simulink model "QPSK_system_v3g"  (R2012b)
settings: Solver=FixedStepDiscrete  SolverMode=SingleTasking  StartTime=0.0  StopTime=6000  FixedStep=1  RelTol=1e-3
libraries: simulink x30, dspsigops x2, dspbuff3 x1, dspsrcs4 x1
(part 4 of 4)

== matlab function QPSK_system_v3g/RX_CORE_TOP/RX/rx_double/qpsk_rx ==
  data: i_in input; byte_out output; q_in input; mu_foc_in input; mu_toc_in input; mcu_rx_ready_in input; en_out output; clear_fifo_out output; num_bytes_ready_out output; r_out output; s_f_out output; s_c_out output; s_t_out output; t_est_out output; s_p_out output; s_o_out output; fe_out output
%%%%%%%%%%%%%%%%%%%%%%%%%%%%%%%%%%%%%%%%%%%%%%%%%%%%%%%%%%%%%%%%%%%%%%%%%%%
% QPSK demonstration packet-based transceiver for Chilipepper
% Toyon Research Corp.
% http://www.toyon.com/chilipepper.php
% Created 10/17/2012
% embedded@toyon.com
%%%%%%%%%%%%%%%%%%%%%%%%%%%%%%%%%%%%%%%%%%%%%%%%%%%%%%%%%%%%%%%%%%%%%%%%%%%
% This file is the top level entry function for the receiver portion of the
% example. The entire receiver is designed to run at Rate=1 (one clock
% cycle per iteration of the core. 
% We follow standard receive practice with frequency offset estimation,
% pulse-shape filtering, time estimateion, and correlation to determine
% tart of packet.
%%%%%%%%%%%%%%%%%%%%%%%%%%%%%%%%%%%%%%%%%%%%%%%%%%%%%%%%%%%%%%%%%%%%%%%%%%%
%#codegen
function [byte_out, en_out, clear_fifo_out, num_bytes_ready_out, ...
        r_out, s_f_out, s_c_out, s_t_out, t_est_out, s_p_out, s_o_out, ...
        fe_out] = ...
    qpsk_rx(i_in, q_in, mu_foc_in, mu_toc_in, mcu_rx_ready_in)

persistent finish_rx_latch

if isempty(finish_rx_latch)
    finish_rx_latch = 0; % feedback once packet is received to rest
end

i_in = round(i_in);
q_in = round(q_in);

% scale input data coming from the Chilipepper ADC to be purely fractional
% to avoid scaling issues
r_in = complex(i_in, q_in);

% frequency offset estimation. Note that time constant is input as integer
[s_f_i, s_f_q, fe] = ...
    qpsk_rx_foc(i_in, q_in, mu_foc_in, finish_rx_latch);

   if finish_rx_latch > 0
    a=0;
   end

% Square-root raised-cosine band-limited filtering
[s_c_i, s_c_q] = qpsk_rx_srrc(s_f_i, s_f_q);

% Time offset estimation. Output data changes at the symbol rate.
[s_t_i, s_t_q, tauh] = ...
    qpsk_rx_toc(s_c_i, s_c_q, mu_toc_in, finish_rx_latch);

% Determine start of packet using front-loaded training sequence
[byte, en, finish_rx, clear_fifo, num_bytes_ready_out, s_p, s_o] = ...
    qpsk_rx_correlator(s_t_i, s_t_q, mcu_rx_ready_in);


% These are debug outputs and can largely be ignored as they are just used
% for testbench simulation
byte_out = byte;
en_out = en;
clear_fifo_out = clear_fifo;

finish_rx_latch = finish_rx;

%r_out = real(r_in);
r_out = r_in;
s_f_out = complex(s_f_i,s_f_q);
s_c_out = complex(s_c_i,s_c_q);
s_t_out = complex(s_t_i,s_t_q);

t_est_out = tauh;
s_p_out = s_p;
s_o_out = s_o;
fe_out = fe;

== matlab function QPSK_system_v3g/RX_CORE_TOP/RX/rx_double/dc_offset ==
  data: i_in input; i_out output; q_in input; alpha_in input; gain_en_in input; rssi_low_goal_in input; rssi_high_goal_in input; rx_en_in input; q_out output; rssi_out output; rssi_en_out output; dir_out output; dir_en_out output; d1 output; d2 output; d3 output; d4 output; d5 output; d6 output; d7 output; d8 output; d9 output
function [i_out, q_out, rssi_out, rssi_en_out, dir_out, dir_en_out, ...
    d1, d2, d3, d4, d5, d6, d7, d8, d9] = ...
    dc_offset_correction(i_in, q_in, alpha_in, gain_en_in, ...
        rssi_low_goal_in, rssi_high_goal_in, rx_en_in)

persistent i_dc q_dc i_mean q_mean
persistent counter rssi_sum
persistent dir_state
persistent rssiHold
persistent noise_offset noise_inc noise_dec

alpha = alpha_in/2^12;

if isempty(i_dc)
    i_dc = 0;
    q_dc = 0;
    i_mean = 0;
    q_mean = 0;
    counter = 0;
    noise_inc = 0;
    noise_dec = 0;
    noise_offset = 0;
    rssi_sum = 0;
    dir_state = 0;
    rssiHold = 0;
end

%%%%%%%%%%%%%%%%%%%%%%%%%%%%%%%%%%%%%%%%%%%%%%%%%%%%%%%%%%%%%%%%%%%%%%%%%%%
% DC Correction section
%%%%%%%%%%%%%%%%%%%%%%%%%%%%%%%%%%%%%%%%%%%%%%%%%%%%%%%%%%%%%%%%%%%%%%%%%%%
if rx_en_in == 1
    i_mean = (1-alpha)*i_mean + alpha*i_in;
    q_mean = (1-alpha)*q_mean + alpha*q_in;

    i_dc = (1-alpha)*i_dc + alpha*i_in; %update the i dc offset
    q_dc = (1-alpha)*q_dc + alpha*q_in; %update the q dc offset

    if abs(i_mean) > (50 + noise_offset)  % too much noise, raise cieling.
        noise_inc = noise_inc + 1;
        i_dc = 0;
    else
        noise_dec = noise_dec + 1;
    end
    if abs(q_mean) > (50 + noise_offset)  % too much noise, raise cieling.
        noise_inc = noise_inc + 1;
        q_dc = 0;
    else
        noise_dec = noise_dec +1;
    end
    if (noise_inc > 10)
        %there is a high dc_offset value that needs to be corrected
        noise_offset = noise_offset + 10;
        noise_inc = 0;
    end
    if (noise_dec > 100000)
        %dc offset threshold is higher than needed
        noise_offset = noise_offset - 10;
        noise_dec = 0;
    end
end
i_out = i_in - i_dc;
q_out = q_in - q_dc;
%correct false positive/nagatives
if (abs(i_mean) < 50)
    noise_inc = 0;
end
if (abs(i_mean) > noise_offset - 10)
    noise_dec = 0;
end
%%%%%%%%%%%%%%%%%%%%%%%%%%%%%%%%%%%%%%%%%%%%%%%%%%%%%%%%%%%%%%%%%%%%%%%%%%%

%%%%%%%%%%%%%%%%%%%%%%%%%%%%%%%%%%%%%%%%%%%%%%%%%%%%%%%%%%%%%%%%%%%%%%%%%%%
% RSSI Estimation
%%%%%%%%%%%%%%%%%%%%%%%%%%%%%%%%%%%%%%%%%%%%%%%%%%%%%%%%%%%%%%%%%%%%%%%%%%%
rssi_inst = i_out*i_out + q_out*q_out;
rssi_en_out = 0;
rssi_out = 0;

if rx_en_in == 1
    if counter == 0 && rssi_inst > 2*50*50
        counter = 1;
        rssi_sum = 0;
    end

    if counter ~= 0
        if rssi_inst < 2*50*50
            counter = 0;
        else
            counter = counter + 1;
            rssi_sum = rssi_sum + rssi_inst;

            if counter >= 2^8
                counter = 0;
                rssi_out = round(rssi_sum/2^8);
                rssiHold = rssi_out;
                rssi_en_out = 1;
            end
        end
    end
end
%%%%%%%%%%%%%%%%%%%%%%%%%%%%%%%%%%%%%%%%%%%%%%%%%%%%%%%%%%%%%%%%%%%%%%%%%%%
   
%%%%%%%%%%%%%%%%%%%%%%%%%%%%%%%%%%%%%%%%%%%%%%%%%%%%%%%%%%%%%%%%%%%%%%%%%%%
% Gain Correction
%%%%%%%%%%%%%%%%%%%%%%%%%%%%%%%%%%%%%%%%%%%%%%%%%%%%%%%%%%%%%%%%%%%%%%%%%%%
dir_out = 0;
dir_en_out = 0;

% dir_out = 0 - do nothing
% dir_out = 1 - increase
% dir_out = 2 - decrease
ai = abs(i_in);
aq = abs(q_in);
% only increase power if the rssi is away from the mean
rssi_diff = abs(rssiHold-(i_mean*i_mean+q_mean*q_mean));
if rx_en_in == 1
    switch dir_state
        case 0 % wait for some action and the processor is done
            if gain_en_in == 0
                if rssi_en_out == 1
                    if rssi_diff < rssi_low_goal_in %too low - increase
                        dir_out = 1;
                        dir_en_out = 1;
                        dir_state = 1;
                    end
                    if rssi_diff > rssi_high_goal_in %too high - decrease
                        dir_out = 2;
                        dir_en_out = 1;
                        dir_state = 1;
                    end
                end
                % we're saturating the ADC so decrease gain
                % this overrides anything else
                if (ai > 1500) || (aq > 1500) 
                    dir_out = 2; % decrease
                    dir_en_out = 1;
                    dir_state = 1;
                end
            end
        case 1 % see if the MCU has done something and if so reset
            if gain_en_in == 1
                dir_out = 0;
                dir_en_out = 1;
                dir_state = 0;
            end
        otherwise
            dir_state = 0;
    end
end
d1 = i_in;
d2 = i_mean;
d3 = i_dc;
d4 = rssiHold;
d5 = rssi_diff;
d6 = dir_state;
d7 = gain_en_in;
d8 = dir_out;
d9 = dir_en_out;
%%%%%%%%%%%%%%%%%%%%%%%%%%%%%%%%%%%%%%%%%%%%%%%%%%%%%%%%%%%%%%%%%%%%%%%%%%%

== matlab function QPSK_system_v3g/FIFO_RX/print/MATLAB Function ==
  data: byte_in input
function  fcn(byte_in)
coder.extrinsic('native2unicode')
persistent index_mess
persistent RecBytes

if isempty(index_mess)
    index_mess = 1;
    RecBytes = zeros(1,18);
end 

if mod(index_mess,2) == 0
    RecBytes(index_mess/2) = byte_in;
end

index_mess = index_mess+1;

if RecBytes(18) > 0
    numRecBytes = RecBytes(1)+RecBytes(2)+RecBytes(3);
    msgBytes = RecBytes((1+4):(numRecBytes+4));
    Message_Received_fixed = native2unicode(msgBytes)
end
